simulink model "AircraftSimulation_RealTime"  (R2017a)
settings: Solver=ode45  StartTime=0.0  StopTime=inf  RelTol=1e-3  EnableMultiTasking=on
model workspace (MAT data in the model file):
  rho = Simulink.Parameter
  rho.Value = 1.225
  rho.DataType = 'auto'
  rho.Dimensions = [1 1]
values from neighbouring files (symbols this model uses):
  AR = 9.8    [ControlTuning.m]
  b = 12.8016    [ControlTuning.m]
  c = 1.3533    [ControlTuning.m]
  D = d    [rscale.m]
  m = 2521    [ControlTuning.m]
  N = inv([A,B;C,D])*Z'    [rscale.m]
  rho = 0.66    [ControlTuning.m]
  S = 16.72254    [ControlTuning.m]
  s = tf('s')    [ControlTuning.m]    (also in rscale.m = size(A,1))
  W = m*g    (= 24731.01)    [ControlTuning.m]
  Z = [zeros([1,s]) 1]    [rscale.m]
  zeta = Ix*Iz - Ixz^2    (= 5250689.81)    [ControlTuning.m]
undefined symbols (not defined in the file or in its folder): cdo, CLa, ClB, Clda, CLde, Cldr, CLmax, CLo, Clp, CLq, Clr, Cma, Cmde, Cmo, Cmq, CnB, Cnda, Cndr, Cnp, Cnr, CYB, CYda, CYdr, CYp, CYr, da, de, dr, dT, dV_x, dV_y, dV_z, elevation, h, I, Isp, mo, mu_e, springK, StallAngle, T, tblackstrip, tControl, tWind, X, xground, xland, Y, yground, yland, ZeroTolerance
libraries: sm_lib x46, nesl_utility x21, simulink x10, realtime_pacer_lib x1
(part 1 of 2)
settings Model: Creator=alexandermclean  LastModifiedBy=alexandermclean
settings SolverCC: ZeroCrossAlgorithm=Adaptive
settings DataIOCC: LimitDataPoints=on  MaxDataPoints=3000  SaveFormat=Array  SaveState=on  ReturnWorkspaceOutputs=on
settings OptimizationCC: LifeSpan=inf
settings DebuggingCC: SFUnexpectedBacktrackingDiag=warning  SFNoUnconditionalDefaultTransitionDiag=warning  SFExecutionAtInitializationDiag=none
settings HardwareCC: ProdBitPerPointer=32  ProdBitPerSizeT=32  ProdBitPerPtrDiffT=32  ProdLargestAtomicFloat=None  ProdIntDivRoundTo=Undefined  ProdEndianess=Unspecified  ProdWordSize=32  ProdHWDeviceType=32-bit Generic
settings ModelReferenceCC: PropagateSignalLabelsOutOfModel=off
settings GRTTargetCC: TargetLangStandard=C89/C90 (ANSI)  GeneratePreprocessorConditionals=Disable all
settings ConfigComp: CovMetricSettings=dw  CovHtmlReporting=on  CovSaveCumulativeToWorkspaceVar=on  CovSaveSingleToWorkspaceVar=on  CovExternalEMLEnable=off
settings ExplorerConfigSet: InternalSimMechanicsExplorerSettings="<ExplorerConfiguration><canonicalview>default</canonicalview><AnimationSetting><BasePlaybackSpeed>1.0</BasePlaybackSpeed><PlaybackSpeedFactor>1.0</PlaybackSpeedFactor></AnimationSetting><TilePanel><TileInfo><Tiles Columns=\"1\" Count=\"1\" Rows=\"1\"><Column Left=\"2\" Weight=\"1\"/><Column Left=\"358\"/><Row Top=\"2\" Weight=\"1\"/><Row Top=\"515\"/><Tile Height=\"1\" Width=\"1\" X=\"0\" Y=\"0\"/></Tiles></TileInfo><SceneInfo><SceneViewer><BGColor><R>0.200000002980232239</R><G>1</G><B>1</B></BGColor><Camera><DoPerspective>off</DoPerspective><Position><X>-5383371.51956753805</X><Y>16528461.3354325853</Y><Z>-20295565.3065634556</Z></Position><Center><X>-424001.534646867425</X><Y>1302358.08165564947</Y><Z>-1688034.52349125012</Z></Center><Up><X>0.659279124000458405</X><Y>-0.486194351728896135</Y><Z>-0.573555654670152237</Z></Up><ViewLimDist>1</ViewLimDist><YLim>4.3662398520704988e-10</YLim><XLim>3.00612148545329968e-10</XLim></Camera></SceneViewer></SceneInfo></TilePanel><MechEditorPanel><Cameras><Camera><Id>Camera1</Id><Value><Name>Driver View</Name><NativeCamera><PositionTrackingFeature>Aircraft_Simulation.Dynamics_Simscape.Drivers_View1.R</PositionTrackingFeature><CenterTrackingFeature>Aircraft_Simulation.Dynamics_Simscape.Drivers_View1.R</CenterTrackingFeature><UpVectorTrackingFeature>Aircraft_Simulation.Dynamics_Simscape.Drivers_View1.R</UpVectorTrackingFeature><CenterTrackingOrigin>off</CenterTrackingOrigin><CenterTrackingDirection>+X</CenterTrackingDirection><UpVectorTrackingDirection>+Z</UpVectorTrackingDirection></NativeCamera></Value></Camera><Camera><Id>Camera2</Id><Value><Name>Front View</Name><NativeCamera><PositionTrackingFeature>Aircraft_Simulation.Dynamics_Simscape.Front_View1.R</PositionTrackingFeature><CenterTrackingFeature>Aircraft_Simulation.Dynamics_Simscape.Front_View1.R</CenterTrackingFeature><UpVectorTrackingFeature>Aircraft_Simulation.Dynamics_Simscape.Front_View1.R</UpVectorTrackingFeature><CenterTrackingOrigin>off</CenterTrackingOrigin><CenterTrackingDirection>-Z</CenterTrackingDirection><UpVectorTrackingDirection>-X</UpVectorTrackingDirection></NativeCamera></Value></Camera><Camera><Id>Camera3</Id><Value><Name>Side View</Name><NativeCamera><PositionTrackingFeature>Aircraft_Simulation.Dynamics_Simscape.Side_View1.R</PositionTrackingFeature><CenterTrackingFeature>Aircraft_Simulation.Dynamics_Simscape.Side_View1.R</CenterTrackingFeature><UpVectorTrackingFeature>Aircraft_Simulation.Dynamics_Simscape.Side_View1.R</UpVectorTrackingFeature><CenterTrackingOrigin>off</CenterTrackingOrigin><CenterTrackingDirection>+Y</CenterTrackingDirection><UpVectorTrackingDirection>-X</UpVectorTrackingDirection></NativeCamera></Value></Camera></Cameras><GfxPanelCameraMap/><VideoCreator><PlaybackSpeedRatio>1.0</PlaybackSpeedRatio><FrameRate>30</FrameRate><VideoFormat>Motion JPEG AVI</VideoFormat><FrameSize>auto</FrameSize></VideoCreator></MechEditorPanel></ExplorerConfiguration>"

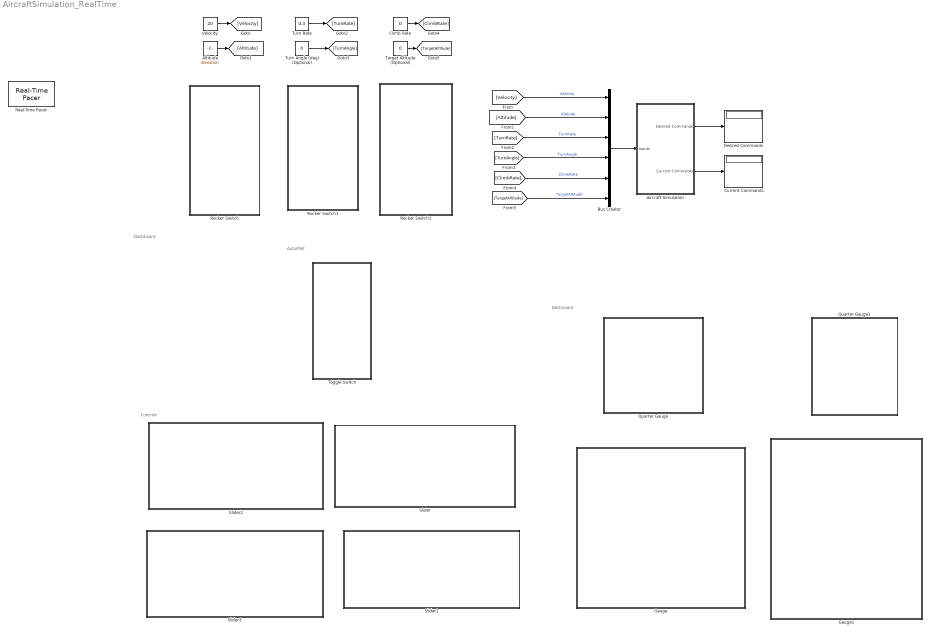
== system AircraftSimulation_RealTime ==
  note: Dashboard
  note: Controls
  note: Dashnoard
  note: AutoPilot
  Aircraft Simulation : Subsystem
  Altitude : Constant  Value=elevation
  Bus Creator : BusCreator  Inputs=6
  Climb Rate : Constant  Value=0
  Current Commands : Display
  Desired Commands : Display
  Gauge : Subsystem  DialogController=hmiCreateDDGDialog  IsWebBlock=on  mask(MWDashboardBlock){webBlockId=67f8af45-a9bd-4350-b479-67b86532381e, webBlockType=circulargauge, ShowInLibBrowser=on, ShowInitialText=on, HMISrcModelName=AircraftSimulation_RealTime}
      mask prompts: webBlockId "WebBlock Id"; webBlockType "WebBlock Type"; HMISrcModelName "Source Model"
      mask help: SimulinkHMI:dialogs:CircularGaugeDialogDesc
      mask Help: helpview([docroot '/mapfiles/simulink.map'], 'hmi_gauge')
      mask Display:
      | if strcmp(get_param(bdroot(gcb),'BlockDiagramType'), 'library')
      |     image([(matlabroot) '/toolbox/simulink/hmi/icons/CircularGauge.png']);
      | end
  Gauge1 : Subsystem  DialogController=hmiCreateDDGDialog  IsWebBlock=on  mask(MWDashboardBlock){webBlockId=380ac432-086c-412e-99f4-435f69615b16, webBlockType=circulargauge, ShowInLibBrowser=on, ShowInitialText=on, HMISrcModelName=AircraftSimulation_RealTime}
      mask prompts: webBlockId "WebBlock Id"; webBlockType "WebBlock Type"; HMISrcModelName "Source Model"
      mask help: SimulinkHMI:dialogs:CircularGaugeDialogDesc
      mask Help: helpview([docroot '/mapfiles/simulink.map'], 'hmi_gauge')
      mask Display:
      | if strcmp(get_param(bdroot(gcb),'BlockDiagramType'), 'library')
      |     image([(matlabroot) '/toolbox/simulink/hmi/icons/CircularGauge.png']);
      | end
  Quarter Gauge : Subsystem  DialogController=hmiCreateDDGDialog  IsWebBlock=on  mask(MWDashboardBlock){webBlockId=95437b06-cebb-4a55-906e-b2c61c378e79, webBlockType=ninetydegreegauge, ShowInLibBrowser=on, ShowInitialText=on, HMISrcModelName=AircraftSimulation_RealTime}
      mask prompts: webBlockId "WebBlock Id"; webBlockType "WebBlock Type"; HMISrcModelName "Source Model"
      mask help: SimulinkHMI:dialogs:NinetydegreeGaugeDialogDesc
      mask Help: helpview([docroot '/mapfiles/simulink.map'], 'hmi_quarter_gauge')
      mask Display:
      | if strcmp(get_param(bdroot(gcb),'BlockDiagramType'), 'library')
      |     image([(matlabroot) '/toolbox/simulink/hmi/icons/NinetyDegreeGauge.png']);
      | end
  Quarter Gauge1 : Subsystem  DialogController=hmiCreateDDGDialog  IsWebBlock=on  mask(MWDashboardBlock){webBlockId=bd2f9303-b0cf-4f11-bfc9-0c1a96ff53ef, webBlockType=ninetydegreegauge, ShowInLibBrowser=on, ShowInitialText=on, HMISrcModelName=AircraftSimulation_RealTime}
      mask prompts: webBlockId "WebBlock Id"; webBlockType "WebBlock Type"; HMISrcModelName "Source Model"
      mask help: SimulinkHMI:dialogs:NinetydegreeGaugeDialogDesc
      mask Help: helpview([docroot '/mapfiles/simulink.map'], 'hmi_quarter_gauge')
      mask Display:
      | if strcmp(get_param(bdroot(gcb),'BlockDiagramType'), 'library')
      |     image([(matlabroot) '/toolbox/simulink/hmi/icons/NinetyDegreeGauge.png']);
      | end
  Real-Time Pacer : realtime_pacer_lib/Real-Time Pacer  simTimePerRealTime=1
  Rocker Switch : Subsystem  DialogController=hmiCreateDDGDialog  IsWebBlock=on  mask(MWDashboardBlock){webBlockId=fc3eccde-041d-4b84-9ecd-21842f4d67ff, webBlockType=rockerswitch, ShowInLibBrowser=on, ShowInitialText=on, HMISrcModelName=AircraftSimulation_RealTime}
      mask prompts: webBlockId "WebBlock Id"; webBlockType "WebBlock Type"; HMISrcModelName "Source Model"
      mask help: SimulinkHMI:dialogs:SwitchDialogDesc
      mask Help: helpview([docroot '/mapfiles/simulink.map'], 'hmi_rocker_switch')
      mask Display:
      | if strcmp(get_param(bdroot(gcb),'BlockDiagramType'), 'library')
      |     image([(matlabroot) '/toolbox/simulink/hmi/icons/RockerSwitch.png']);
      | end
  Rocker Switch1 : Subsystem  DialogController=hmiCreateDDGDialog  IsWebBlock=on  mask(MWDashboardBlock){webBlockId=dc990da5-677e-4d98-94b9-87c965764d26, webBlockType=rockerswitch, ShowInLibBrowser=on, ShowInitialText=on, HMISrcModelName=AircraftSimulation_RealTime}
      mask prompts: webBlockId "WebBlock Id"; webBlockType "WebBlock Type"; HMISrcModelName "Source Model"
      mask help: SimulinkHMI:dialogs:SwitchDialogDesc
      mask Help: helpview([docroot '/mapfiles/simulink.map'], 'hmi_rocker_switch')
      mask Display:
      | if strcmp(get_param(bdroot(gcb),'BlockDiagramType'), 'library')
      |     image([(matlabroot) '/toolbox/simulink/hmi/icons/RockerSwitch.png']);
      | end
  Rocker Switch2 : Subsystem  DialogController=hmiCreateDDGDialog  IsWebBlock=on  mask(MWDashboardBlock){webBlockId=1b32aaf5-d39d-42dc-bc83-2804a198291e, webBlockType=rockerswitch, ShowInLibBrowser=on, ShowInitialText=on, HMISrcModelName=AircraftSimulation_RealTime}
      mask prompts: webBlockId "WebBlock Id"; webBlockType "WebBlock Type"; HMISrcModelName "Source Model"
      mask help: SimulinkHMI:dialogs:SwitchDialogDesc
      mask Help: helpview([docroot '/mapfiles/simulink.map'], 'hmi_rocker_switch')
      mask Display:
      | if strcmp(get_param(bdroot(gcb),'BlockDiagramType'), 'library')
      |     image([(matlabroot) '/toolbox/simulink/hmi/icons/RockerSwitch.png']);
      | end
  Slider : Subsystem  DialogController=hmiCreateDDGDialog  IsWebBlock=on  mask(MWDashboardBlock){webBlockId=21ec2cde-896d-490e-83b9-19082907d4f5, webBlockType=slider, ShowInLibBrowser=on, ShowInitialText=on, HMISrcModelName=AircraftSimulation_RealTime}
      mask prompts: webBlockId "WebBlock Id"; webBlockType "WebBlock Type"; HMISrcModelName "Source Model"
      mask help: SimulinkHMI:dialogs:SliderDialogDesc
      mask Help: helpview([docroot '/mapfiles/simulink.map'], 'hmi_slider')
      mask Display:
      | if strcmp(get_param(bdroot(gcb),'BlockDiagramType'), 'library')
      |     image([(matlabroot) '/toolbox/simulink/hmi/icons/Slider.png']);
      | end
  Slider1 : Subsystem  DialogController=hmiCreateDDGDialog  IsWebBlock=on  mask(MWDashboardBlock){webBlockId=1d21c48f-609f-4438-ac6a-622a61b7def2, webBlockType=slider, ShowInLibBrowser=on, ShowInitialText=on, HMISrcModelName=AircraftSimulation_RealTime}
      mask prompts: webBlockId "WebBlock Id"; webBlockType "WebBlock Type"; HMISrcModelName "Source Model"
      mask help: SimulinkHMI:dialogs:SliderDialogDesc
      mask Help: helpview([docroot '/mapfiles/simulink.map'], 'hmi_slider')
      mask Display:
      | if strcmp(get_param(bdroot(gcb),'BlockDiagramType'), 'library')
      |     image([(matlabroot) '/toolbox/simulink/hmi/icons/Slider.png']);
      | end
  Slider2 : Subsystem  DialogController=hmiCreateDDGDialog  IsWebBlock=on  mask(MWDashboardBlock){webBlockId=c2aec1fe-8232-42fd-811c-b469951ff54e, webBlockType=slider, ShowInLibBrowser=on, ShowInitialText=on, HMISrcModelName=AircraftSimulation_RealTime}
      mask prompts: webBlockId "WebBlock Id"; webBlockType "WebBlock Type"; HMISrcModelName "Source Model"
      mask help: SimulinkHMI:dialogs:SliderDialogDesc
      mask Help: helpview([docroot '/mapfiles/simulink.map'], 'hmi_slider')
      mask Display:
      | if strcmp(get_param(bdroot(gcb),'BlockDiagramType'), 'library')
      |     image([(matlabroot) '/toolbox/simulink/hmi/icons/Slider.png']);
      | end
  Slider3 : Subsystem  DialogController=hmiCreateDDGDialog  IsWebBlock=on  mask(MWDashboardBlock){webBlockId=bc4d324b-da30-4baa-91b4-3aa56de8667c, webBlockType=slider, ShowInLibBrowser=on, ShowInitialText=on, HMISrcModelName=AircraftSimulation_RealTime}
      mask prompts: webBlockId "WebBlock Id"; webBlockType "WebBlock Type"; HMISrcModelName "Source Model"
      mask help: SimulinkHMI:dialogs:SliderDialogDesc
      mask Help: helpview([docroot '/mapfiles/simulink.map'], 'hmi_slider')
      mask Display:
      | if strcmp(get_param(bdroot(gcb),'BlockDiagramType'), 'library')
      |     image([(matlabroot) '/toolbox/simulink/hmi/icons/Slider.png']);
      | end
  Target Altitude (Optional) : Constant  Value=0
  Toggle Switch : Subsystem  DialogController=hmiCreateDDGDialog  IsWebBlock=on  mask(MWDashboardBlock){webBlockId=dcb6ed43-b1b9-4957-aceb-26a4fc5c1c0a, webBlockType=toggleswitch, ShowInLibBrowser=on, ShowInitialText=on, HMISrcModelName=AircraftSimulation_RealTime}
      mask prompts: webBlockId "WebBlock Id"; webBlockType "WebBlock Type"; HMISrcModelName "Source Model"
      mask help: SimulinkHMI:dialogs:SwitchDialogDesc
      mask Help: helpview([docroot '/mapfiles/simulink.map'], 'hmi_toggle_switch')
      mask Display:
      | if strcmp(get_param(bdroot(gcb),'BlockDiagramType'), 'library')
      |     image([(matlabroot) '/toolbox/simulink/hmi/icons/ToggleSwitch.png']);
      | end
  "Turn Angle (deg) (Optional) " : Constant  Value=0
  Turn Rate : Constant  Value=0.3
  Velocity : Constant  Value=20
  wires:
  Aircraft Simulation/1(Desired Commands) -> Desired Commands/1
  Aircraft Simulation/2(Current Commands) -> Current Commands/1
  Bus Creator/1 -> Aircraft Simulation/1(Inputs)
  Velocity/1 -> [Velocity]
  Altitude/1 -> [Altitude]
  Turn Rate/1 -> [TurnRate]
  "Turn Angle (deg) (Optional) "/1 -> [TurnAngle]
  Climb Rate/1 -> [ClimbRate]
  Target Altitude (Optional)/1 -> [TargetAltitude]
  [Velocity] -> Bus Creator/1  "Velocity"
  [Altitude] -> Bus Creator/2  "Altitude"
  [TurnRate] -> Bus Creator/3  "TurnRate"
  [TurnAngle] -> Bus Creator/4  "TurnAngle"
  [ClimbRate] -> Bus Creator/5  "ClimbRate"
  [TargetAltitude] -> Bus Creator/6  "TargetAltitude"

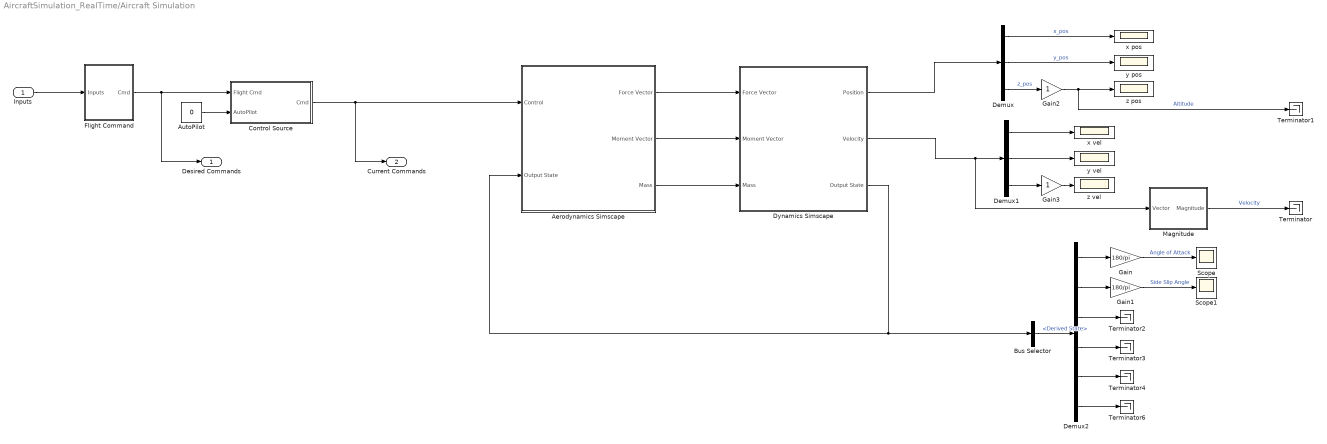
== system AircraftSimulation_RealTime/Aircraft Simulation ==
  Inputs : Inport
  Aerodynamics Simscape : Subsystem
  AutoPilot : Constant  Value=0
  Bus Selector : BusSelector  OutputSignals=Derived State
  Control Source : Subsystem
  Demux : Demux  Outputs=3
  Demux1 : Demux  Outputs=3
  Demux2 : Demux  Outputs=6
  Dynamics Simscape : Subsystem
  Flight Command : Subsystem
  Gain : Gain  Gain=180/pi
  Gain1 : Gain  Gain=180/pi
  Gain2 : Gain
  Gain3 : Gain
  Magnitude : Subsystem
  Scope : Scope
  Scope1 : Scope
  Terminator{,1..4,6} (6 alike) : Terminator
  x pos : Scope
  x vel : Scope
  y pos : Scope
  y vel : Scope
  z pos : Scope
  z vel : Scope
  Desired Commands : Outport
  Current Commands : Outport  Port=2
  wires:
  Magnitude/1(Magnitude) -> Terminator/1  "Velocity"
  Aerodynamics Simscape/1(Force Vector) -> Dynamics Simscape/1(Force Vector)
  Aerodynamics Simscape/2(Moment Vector) -> Dynamics Simscape/2(Moment Vector)
  AutoPilot/1 -> Control Source/2(AutoPilot)
  Control Source/1(Cmd) -> Current Commands/1, Aerodynamics Simscape/1(Control)
  Flight Command/1(Cmd) -> Desired Commands/1, Control Source/1(Flight Cmd)
  Demux/1 -> x pos/1  "x_pos"
  Demux/2 -> y pos/1  "y_pos"
  Demux/3 -> Gain2/1  "z_pos"
  Dynamics Simscape/3(Output State) -> Aerodynamics Simscape/2(" Output State"), Bus Selector/1
  Aerodynamics Simscape/3(Mass) -> Dynamics Simscape/3(Mass)
  Demux1/3 -> Gain3/1
  Demux1/1 -> x vel/1
  Dynamics Simscape/2(Velocity) -> Magnitude/1(Vector), Demux1/1
  Demux1/2 -> y vel/1
  Demux2/6 -> Terminator6/1
  Demux2/3 -> Terminator2/1
  Demux2/1 -> Gain/1
  Demux2/2 -> Gain1/1
  Demux2/4 -> Terminator3/1
  Dynamics Simscape/1(Position) -> Demux/1
  Bus Selector/1 -> Demux2/1  "<Derived State>"
  Demux2/5 -> Terminator4/1
  Gain1/1 -> Scope1/1  "Side Slip Angle"
  Gain/1 -> Scope/1  "Angle of Attack"
  Inputs/1 -> Flight Command/1(Inputs)
  Gain2/1 -> Terminator1/1, z pos/1  "Altitude"
  Gain3/1 -> z vel/1

== system AircraftSimulation_RealTime/Gauge ==

== system AircraftSimulation_RealTime/Gauge1 ==

== system AircraftSimulation_RealTime/Quarter Gauge ==

== system AircraftSimulation_RealTime/Quarter Gauge1 ==

== system AircraftSimulation_RealTime/Rocker Switch ==

== system AircraftSimulation_RealTime/Rocker Switch1 ==

== system AircraftSimulation_RealTime/Rocker Switch2 ==

== system AircraftSimulation_RealTime/Slider ==

== system AircraftSimulation_RealTime/Slider1 ==

== system AircraftSimulation_RealTime/Slider2 ==

== system AircraftSimulation_RealTime/Slider3 ==

== system AircraftSimulation_RealTime/Toggle Switch ==

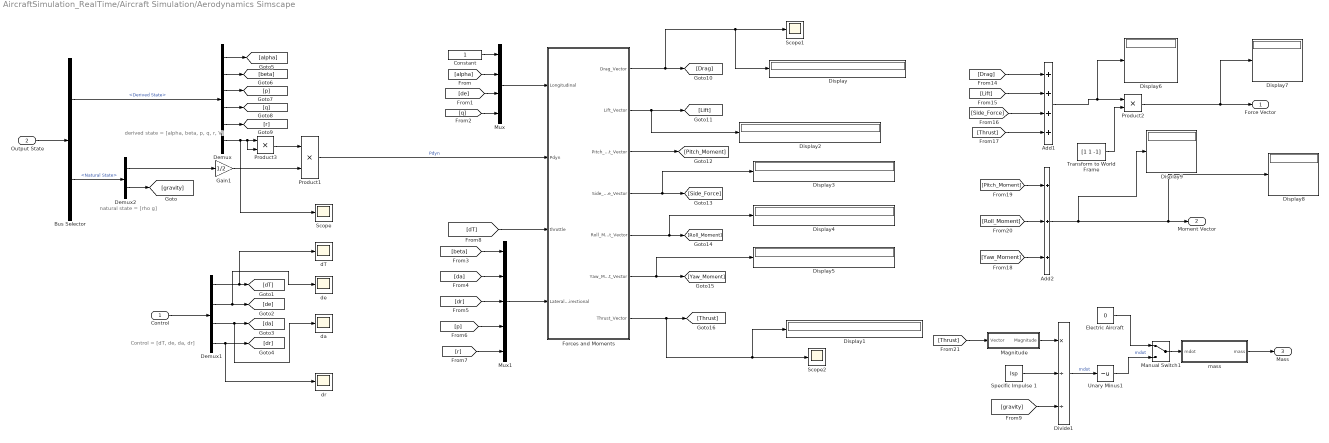
== system AircraftSimulation_RealTime/Aircraft Simulation/Aerodynamics Simscape ==
  note: Control = [dT, de, da, dr]
  note: derived state = [alpha, beta, p, q, r, V]
  note: natural state = [rho g]
  Control : Inport
  " Output State" : Inport  Port=2
  Add1 : Sum  Inputs=++++
  Add2 : Sum  Inputs=+++
  Bus Selector : BusSelector  OutputSignals=Derived State,Natural State
  Constant : Constant
  Demux : Demux  Outputs=6
  Demux1 : Demux
  Demux2 : Demux  Outputs=2
  Display{,1..9} (10 alike) : Display
  Divide1 : Product  Inputs=*//
  Electric Aircraft : Constant  Value=0
  Forces and Moments : Subsystem
  Gain1 : Gain  Gain=1/2
  Magnitude : Subsystem
  Manual Switch1 : ManualSwitch
  Mux : Mux
  Mux1 : Mux  Inputs=5
  Product1 : Product
  Product2 : Product
  Product3 : Product
  Scope : Scope
  Scope1 : Scope
  Scope2 : Scope
  Specific Impulse 1 : Constant  Value=Isp
  Transform to World Frame : Constant  Value=[1 1 -1]
  Unary Minus1 : UnaryMinus
  dT : Scope
  da : Scope
  de : Scope
  dr : Scope
  mass : Subsystem
  Force Vector : Outport
  Moment Vector : Outport  Port=2
  Mass : Outport  Port=3
  wires:
  Demux1/3 -> [da], da/1
  mass/1(mass) -> Mass/1
  Manual Switch1/1 -> mass/1(mdot)
  [dT] -> Forces and Moments/3("throttle ")
  Forces and Moments/7(Thrust_Vector) -> [Thrust], Scope2/1, Display1/1
  Forces and Moments/6(Yaw_Moment_Vector) -> [Yaw_Moment], Display5/1
  Forces and Moments/5(Roll_Moment_Vector) -> [Roll_Moment], Display4/1
  Forces and Moments/4(Side_Force_Vector) -> [Side_Force], Display3/1
  Forces and Moments/3(Pitch_Moment_Vector) -> [Pitch_Moment]
  Forces and Moments/2(Lift_Vector) -> [Lift], Display2/1
  Forces and Moments/1(Drag_Vector) -> [Drag], Scope1/1, Display/1
  Mux1/1 -> Forces and Moments/4(Lateral-Directional)
  Mux/1 -> Forces and Moments/1(Longitudinal)
  Magnitude/1(Magnitude) -> Divide1/1
  [Thrust] -> Magnitude/1(Vector)
  Electric Aircraft/1 -> Manual Switch1/1
  Unary Minus1/1 -> Manual Switch1/2  "mdot"
  [gravity] -> Divide1/3
  Divide1/1 -> Unary Minus1/1  "mdot"
  Specific Impulse 1/1 -> Divide1/2
  [Lift] -> Add1/2
  [Roll_Moment] -> Add2/2
  [Pitch_Moment] -> Add2/1
  [Yaw_Moment] -> Add2/3
  [Thrust] -> Add1/4
  [Side_Force] -> Add1/3
  [Drag] -> Add1/1
  [r] -> Mux1/5
  [beta] -> Mux1/1
  [p] -> Mux1/4
  [dr] -> Mux1/3
  [da] -> Mux1/2
  [q] -> Mux/4
  [de] -> Mux/3
  [alpha] -> Mux/2
  Constant/1 -> Mux/1
  Demux/5 -> [r]
  Demux/4 -> [q]
  Demux/3 -> [p]
  Demux/2 -> [beta]
  Demux/1 -> [alpha]
  Demux1/4 -> [dr], dr/1
  Demux1/2 -> [de], de/1
  Demux1/1 -> [dT], dT/1
  Product1/1 -> Forces and Moments/2(Pdyn)  "Pdyn"
  Gain1/1 -> Product1/2
  Demux2/2 -> [gravity]
  Product3/1 -> Product1/1
  Demux/6 -> Product3/1, Product3/2, Scope/1
  Demux2/1 -> Gain1/1
  Bus Selector/2 -> Demux2/1  "<Natural State>"
  Bus Selector/1 -> Demux/1  "<Derived State>"
  " Output State"/1 -> Bus Selector/1
  Control/1 -> Demux1/1
  Add2/1 -> Display8/1, Moment Vector/1, Display9/1
  Product2/1 -> Display7/1, Force Vector/1
  Transform to World Frame/1 -> Product2/2
  Add1/1 -> Display6/1, Product2/1

== system AircraftSimulation_RealTime/Aircraft Simulation/Control Source ==
  Flight Cmd : Inport
  AutoPilot : Inport  Port=2
  Aileron : Constant  Value=0
  Elevator : Constant  Value=0.0613138686131
  Mux : Mux
  Rudder : Constant  Value=0
  Switch : Switch  Threshold=1
  Thrust : Constant  Value=0
  Cmd : Outport
  wires:
  Switch/1 -> Cmd/1
  AutoPilot/1 -> Switch/2
  Thrust/1 -> Mux/1
  Elevator/1 -> Mux/2
  Rudder/1 -> Mux/4
  Aileron/1 -> Mux/3
  Flight Cmd/1 -> Switch/1
  Mux/1 -> Switch/3

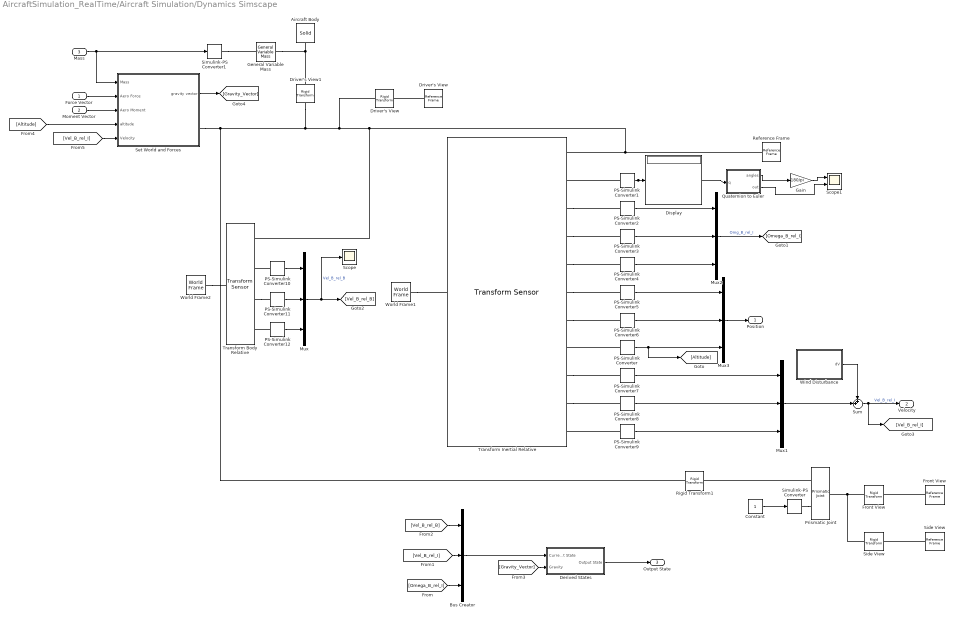
== system AircraftSimulation_RealTime/Aircraft Simulation/Dynamics Simscape ==
  Force Vector : Inport
  Moment Vector : Inport  Port=2
  Mass : Inport  Port=3
  " Driver's View" : sm_lib/Frames and Transforms/Reference Frame
  " Front View" : sm_lib/Frames and Transforms/Reference Frame
  " Side View" : sm_lib/Frames and Transforms/Reference Frame
  Aircraft Body : sm_lib/Body Elements/Solid  InertiaType=Custom  Mass=0  MassUnits=kg  CenterOfMass=[0 0 0]  CenterOfMassUnits=m  MomentsOfInertia=[0 0 0]  MomentsOfInertiaUnits=kg*m^2  ProductsOfInertia=[0 0 0]  ProductsOfInertiaUnits=kg*m^2  DensityBased=off  Density=62.38  DensityUnits=kg/m^3  DoExposeReferenceFrame=on  SerializedFrames=<Frames/>  GraphicType=FromGeometry  MarkerShape=Sphere  MarkerSize=10  GraphicVisPropType=SimpleVisualProperties  GraphicDiffuseColor=[0.5 0.5 0.5]  GraphicSpecularColor=[0.5 0.5 0.5 1.0]  GraphicAmbientColor=[0.15 0.15 0.15 1.0]  GraphicEmissiveColor=[0.0 0.0 0.0 1.0]  GraphicShininess=75  GraphicOpacity=1.0  GeometryShape=FromFile  RectangleSize=[1 1]  RectangleSizeUnits=m  BrickDimensions=[1 1 1]  BrickDimensionUnits=m  CylinderRadius=1  CylinderRadiusUnits=m  CylinderLength=1  CylinderLengthUnits=m  SphereRadius=1  SphereRadiusUnits=m  EllipsoidRadii=[1 1 1]  EllipsoidRadiiUnits=m  ExtrusionCrossSection=[1 1; -1 1; -1 -1; 1 -1]  ExtrusionCrossSectionUnits=m  ExtrusionLength=1  ExtrusionLengthUnits=m  PolygonNumSides=3  PolygonOuterRadius=1  PolygonOuterRadiusUnits=m  ExtGeomFileType=STEP  ExtGeomFileName=/Users/alexandermclean/Documents/MATLAB/BreakPlane/Rc_Aircraft v2.step  ExtGeomFileUnits=m  RevolutionCrossSection=[1 1; 1 -1; 2 -1; 2 1]  RevolutionCrossSectionUnits=m  RevolutionExtent=Full  RevolutionAngle=180  RevolutionAngleUnits=deg
  Bus Creator : BusCreator  Inputs=3
  Constant : Constant
  Derived States : Subsystem
  Display : Display
  Driver's View : sm_lib/Frames and Transforms/Rigid Transform  TranslationMethod=Cartesian  TranslationStandardOffset=0  TranslationLengthUnit=m  TranslationStandardAxis=+Z  TranslationCartesianOffset=driverView  TranslationROffset=0  TranslationROffsetUnits=m  TranslationZOffset=0  TranslationZOffsetUnits=m  TranslationThetaOffset=0  TranslationThetaOffsetUnits=deg  RotationMethod=AlignedAxes  RotationAngleUnits=deg  RotationStandardAxis=+Z  RotationAngle=0.0  RotationArbitraryAxis=[0 0 1]  FollAlignAxisA=+Z  BaseAlignAxisA=-Z  FollAlignAxisB=+X  BaseAlignAxisB=+X  RotationSequenceAxes=FollowerAxes  RotationSequence=XYX  RotationSequenceAngles=[0 0 0]  RotationSequenceAnglesUnits=deg  RotationMatrix=[1 0 0; 0 1 0; 0 0 1]
  Driver's View1 : sm_lib/Frames and Transforms/Rigid Transform  TranslationMethod=Cartesian  TranslationStandardOffset=0  TranslationLengthUnit=m  TranslationStandardAxis=+Z  TranslationCartesianOffset=driverView  TranslationROffset=0  TranslationROffsetUnits=m  TranslationZOffset=0  TranslationZOffsetUnits=m  TranslationThetaOffset=0  TranslationThetaOffsetUnits=deg  RotationMethod=AlignedAxes  RotationAngleUnits=deg  RotationStandardAxis=+Z  RotationAngle=0.0  RotationArbitraryAxis=[0 0 1]  FollAlignAxisA=-X  BaseAlignAxisA=+X  FollAlignAxisB=+Y  BaseAlignAxisB=-Z  RotationSequenceAxes=FollowerAxes  RotationSequence=XYX  RotationSequenceAngles=[0 0 0]  RotationSequenceAnglesUnits=deg  RotationMatrix=[1 0 0; 0 1 0; 0 0 1]
  "Front View " : sm_lib/Frames and Transforms/Rigid Transform  TranslationMethod=Cartesian  TranslationStandardOffset=0  TranslationLengthUnit=m  TranslationStandardAxis=+Z  TranslationCartesianOffset=frontView  TranslationROffset=0  TranslationROffsetUnits=m  TranslationZOffset=0  TranslationZOffsetUnits=m  TranslationThetaOffset=0  TranslationThetaOffsetUnits=deg  RotationMethod=None  RotationAngleUnits=deg  RotationStandardAxis=+Z  RotationAngle=0.0  RotationArbitraryAxis=[0 0 1]  FollAlignAxisA=+Z  BaseAlignAxisA=+X  FollAlignAxisB=+Y  BaseAlignAxisB=+Y  RotationSequenceAxes=FollowerAxes  RotationSequence=XYX  RotationSequenceAngles=[0 0 0]  RotationSequenceAnglesUnits=deg  RotationMatrix=[1 0 0; 0 1 0; 0 0 1]
  Gain : Gain  Gain=180/pi
  General Variable Mass : sm_lib/Body Elements/Variable Mass/General Variable Mass  VariableInertiaType=Custom  MassType=TimeVarying  Mass=1  MassUnits=kg  CenterOfMassType=Constant  CenterOfMass=[h 0 0]  CenterOfMassUnits=m  InertiaMatrixType=Constant  MomentsOfInertia=[I I I]  MomentsOfInertiaUnits=kg*m^2  ProductsOfInertia=[0 0 0]  ProductsOfInertiaUnits=kg*m^2  GraphicType=InertiaEllipsoid  MarkerShape=Sphere  MarkerSize=10  GraphicVisPropType=SimpleVisualProperties  GraphicDiffuseColor=[0 1 0]  GraphicSpecularColor=[0.5 0.5 0.5 1.0]  GraphicAmbientColor=[0.15 0.15 0.15 1.0]  GraphicEmissiveColor=[0.0 0.0 0.0 1.0]  GraphicShininess=75  GraphicOpacity=0
      settings: SourceProductName=Simscape Multibody  SourceProductBaseCode=MS
  Mux{,1..3} (4 alike) : Mux  Inputs=3
  PS-Simulink Converter{,1..12} (13 alike) : nesl_utility/PS-Simulink Converter  PhysicalDomain=network_engine_domain  SubClassName=ps_output  LeftPortType=input  RightPortType=output  PseudoPeriodic=off  Frequencies=[]  Unit=1  AffineConversion=off
  Prismatic Joint : sm_lib/Joints/Prismatic Joint  SenseConstraintForce=off  SenseConstraintForceX=off  SenseConstraintForceY=off  SenseConstraintForceZ=off  SenseConstraintTorque=off  SenseConstraintTorqueX=off  SenseConstraintTorqueY=off  SenseConstraintTorqueZ=off  SenseTotalForce=off  SenseTotalForceX=off  SenseTotalForceY=off  SenseTotalForceZ=off  SenseTotalTorque=off  SenseTotalTorqueX=off  SenseTotalTorqueY=off  SenseTotalTorqueZ=off  CompositeWrenchDir=FollowerOnBase  CompositeWrenchFrame=BaseFrame  EquilibriumPosition=0  EquilibriumPositionUnits=m  SpringStiffness=0  SpringStiffnessUnits=N/m  DampingCoefficient=0  DampingCoefficientUnits=N/(m/s)  TorqueActuationMode=ComputedTorque  MotionActuationMode=InputMotion  SensePosition=off  SenseVelocity=off  SenseAcceleration=off  SenseTorqueForce=off  PositionTargetSpecify=on  PositionTargetPriority=High  PositionTargetValue=0  PositionTargetValueUnits=m  VelocityTargetSpecify=off  VelocityTargetPriority=High  VelocityTargetValue=0  VelocityTargetValueUnits=m/s
  Quaternion to Euler : MATLAB Function  TreatAsAtomicUnit=on
  Reference Frame : sm_lib/Frames and Transforms/Reference Frame
  Rigid Transform1 : sm_lib/Frames and Transforms/Rigid Transform  TranslationMethod=None  TranslationStandardOffset=0  TranslationLengthUnit=m  TranslationStandardAxis=+Z  TranslationCartesianOffset=[0 0 0]  TranslationROffset=0  TranslationROffsetUnits=m  TranslationZOffset=0  TranslationZOffsetUnits=m  TranslationThetaOffset=0  TranslationThetaOffsetUnits=deg  RotationMethod=AlignedAxes  RotationAngleUnits=deg  RotationStandardAxis=+Z  RotationAngle=0.0  RotationArbitraryAxis=[0 0 1]  FollAlignAxisA=+Z  BaseAlignAxisA=-Z  FollAlignAxisB=+Y  BaseAlignAxisB=+Y  RotationSequenceAxes=FollowerAxes  RotationSequence=XZX  RotationSequenceAngles=[90 0 0]  RotationSequenceAnglesUnits=deg  RotationMatrix=[1 0 0; 0 1 0; 0 0 1]
  Scope : Scope
  Scope1 : Scope  NumInputPorts=2
  Set World and Forces : Subsystem
  "Side View " : sm_lib/Frames and Transforms/Rigid Transform  TranslationMethod=Cartesian  TranslationStandardOffset=0  TranslationLengthUnit=m  TranslationStandardAxis=+Z  TranslationCartesianOffset=sideView  TranslationROffset=0  TranslationROffsetUnits=m  TranslationZOffset=0  TranslationZOffsetUnits=m  TranslationThetaOffset=0  TranslationThetaOffsetUnits=deg  RotationMethod=None  RotationAngleUnits=deg  RotationStandardAxis=+Z  RotationAngle=0.0  RotationArbitraryAxis=[0 0 1]  FollAlignAxisA=+Z  BaseAlignAxisA=+X  FollAlignAxisB=+Y  BaseAlignAxisB=+Y  RotationSequenceAxes=FollowerAxes  RotationSequence=XYX  RotationSequenceAngles=[0 0 0]  RotationSequenceAnglesUnits=deg  RotationMatrix=[1 0 0; 0 1 0; 0 0 1]
  Simulink-PS Converter : nesl_utility/Simulink-PS Converter  PhysicalDomain=network_engine_domain  SubClassName=ps_input  LeftPortType=input  RightPortType=output  PseudoPeriodic=off  Frequencies=[]  NoiseDistribution=none  NoiseParameters=[]  Unit=1  AffineConversion=off  FilteringAndDerivatives=provide  SimscapeFilterOrder=1  InputFilterTimeConstant=0.001  UdotUserProvided=0
  Simulink-PS Converter1 : nesl_utility/Simulink-PS Converter  PhysicalDomain=network_engine_domain  SubClassName=ps_input  LeftPortType=input  RightPortType=output  PseudoPeriodic=off  Frequencies=[]  NoiseDistribution=none  NoiseParameters=[]  Unit=1  AffineConversion=off  FilteringAndDerivatives=provide  SimscapeFilterOrder=1  InputFilterTimeConstant=0.001  UdotUserProvided=0
  Sum : Sum  Inputs=++|
  Transform Body Relative : sm_lib/Frames and Transforms/Transform Sensor  MeasurementFrame=NonRotatingFollower  SenseAngle=off  SenseAxis=off  SenseAngle1=off  SenseAngle2=off  SenseAngle3=off  SenseQ=off  SenseR=off  SenseOmegaX=off  SenseOmegaY=off  SenseOmegaZ=off  SenseOmega1=off  SenseOmega2=off  SenseOmega3=off  SenseQDot=off  SenseRDot=off  SenseAlphaX=off  SenseAlphaY=off  SenseAlphaZ=off  SenseAlpha1=off  SenseAlpha2=off  SenseAlpha3=off  SenseQDDot=off  SenseRDDot=off  SenseX=off  SenseY=off  SenseZ=off  SenseRad=off  SenseAzim=off  SenseDist=off  SenseInc=off  SenseXDot=on  SenseYDot=on  SenseZDot=on  SenseRadDot=off  SenseAzimDot=off  SenseDistDot=off  SenseIncDot=off  SenseXDDot=off  SenseYDDot=off  SenseZDDot=off  SenseRadDDot=off  SenseAzimDDot=off  SenseDistDDot=off  SenseIncDDot=off
  Transform Inertial Relative : sm_lib/Frames and Transforms/Transform Sensor  MeasurementFrame=World  SenseAngle=off  SenseAxis=off  SenseAngle1=off  SenseAngle2=off  SenseAngle3=off  SenseQ=on  SenseR=off  SenseOmegaX=on  SenseOmegaY=on  SenseOmegaZ=on  SenseOmega1=off  SenseOmega2=off  SenseOmega3=off  SenseQDot=off  SenseRDot=off  SenseAlphaX=off  SenseAlphaY=off  SenseAlphaZ=off  SenseAlpha1=off  SenseAlpha2=off  SenseAlpha3=off  SenseQDDot=off  SenseRDDot=off  SenseX=on  SenseY=on  SenseZ=on  SenseRad=off  SenseAzim=off  SenseDist=off  SenseInc=off  SenseXDot=on  SenseYDot=on  SenseZDot=on  SenseRadDot=off  SenseAzimDot=off  SenseDistDot=off  SenseIncDot=off  SenseXDDot=off  SenseYDDot=off  SenseZDDot=off  SenseRadDDot=off  SenseAzimDDot=off  SenseDistDDot=off  SenseIncDDot=off
  Wind Disturbance : Subsystem
  World Frame1 : sm_lib/Frames and Transforms/World Frame
  World Frame2 : sm_lib/Frames and Transforms/World Frame
  Position : Outport
  Velocity : Outport  Port=2
  Output State : Outport  Port=3
  wires:
  PS-Simulink Converter5/1 -> Mux3/1
  PS-Simulink Converter6/1 -> Mux3/2
  PS-Simulink Converter8/1 -> Mux1/2
  PS-Simulink Converter7/1 -> Mux1/1
  PS-Simulink Converter2/1 -> Mux2/1
  PS-Simulink Converter3/1 -> Mux2/2
  PS-Simulink Converter4/1 -> Mux2/3
  PS-Simulink Converter1/1 -> Quaternion to Euler/1(q), Display/1
  Force Vector/1 -> Set World and Forces/2(Aero Force)
  Moment Vector/1 -> Set World and Forces/3(Aero Moment)
  PS-Simulink Converter10/1 -> Mux/1
  PS-Simulink Converter11/1 -> Mux/2
  PS-Simulink Converter12/1 -> Mux/3
  Mux/1 -> Scope/1, [Vel_B_rel_B]  "Vel_B_rel_B"
  PS-Simulink Converter9/1 -> Mux1/3
  Mux2/1 -> [Omega_B_rel_I]  "Omg_B_rel_I"
  [Omega_B_rel_I] -> Bus Creator/3
  [Vel_B_rel_I] -> Bus Creator/2
  [Vel_B_rel_B] -> Bus Creator/1
  Bus Creator/1 -> Derived States/1(Current State)
  Set World and Forces/1(gravity vector) -> [Gravity_Vector]
  [Gravity_Vector] -> Derived States/2(Gravity)
  Derived States/1(Output State) -> Output State/1
  [Altitude] -> Set World and Forces/4(altitude)
  Constant/1 -> Simulink-PS Converter/1
  Sum/1 -> [Vel_B_rel_I], Velocity/1  "Vel_B_rel_I"
  Mux1/1 -> Sum/2
  Wind Disturbance/1(dV) -> Sum/1
  Mux3/1 -> Position/1
  Mass/1 -> Set World and Forces/1(Mass), Simulink-PS Converter1/1
  [Vel_B_rel_I] -> Set World and Forces/5(Velocity)
  PS-Simulink Converter/1 -> [Altitude], Mux3/3
  Quaternion to Euler/1(angles) -> Gain/1
  Gain/1 -> Scope1/1
  Quaternion to Euler/2(out) -> Scope1/2
  connections:
  World Frame1/RConn1 -- Transform Inertial Relative/LConn1
  PS-Simulink Converter1/LConn1 -- Transform Inertial Relative/RConn2
  PS-Simulink Converter/LConn1 -- Transform Inertial Relative/RConn8
  PS-Simulink Converter9/LConn1 -- Transform Inertial Relative/RConn11
  Transform Inertial Relative/RConn10 -- PS-Simulink Converter8/LConn1
  Transform Inertial Relative/RConn9 -- PS-Simulink Converter7/LConn1
  Transform Inertial Relative/RConn7 -- PS-Simulink Converter6/LConn1
  Transform Inertial Relative/RConn6 -- PS-Simulink Converter5/LConn1
  Transform Inertial Relative/RConn5 -- PS-Simulink Converter4/LConn1
  Transform Inertial Relative/RConn4 -- PS-Simulink Converter3/LConn1
  Transform Inertial Relative/RConn3 -- PS-Simulink Converter2/LConn1
  World Frame2/RConn1 -- Transform Body Relative/LConn1
  PS-Simulink Converter10/LConn1 -- Transform Body Relative/RConn2
  PS-Simulink Converter12/LConn1 -- Transform Body Relative/RConn4
  Transform Body Relative/RConn3 -- PS-Simulink Converter11/LConn1
  Prismatic Joint/LConn1 -- Rigid Transform1/RConn1
  "Front View "/LConn1 -- "Side View "/LConn1 -- Prismatic Joint/RConn1
  " Side View"/RConn1 -- "Side View "/RConn1
  " Front View"/RConn1 -- "Front View "/RConn1
  " Driver's View"/RConn1 -- Driver's View/RConn1
  Simulink-PS Converter/RConn1 -- Prismatic Joint/LConn2
  Simulink-PS Converter1/RConn1 -- General Variable Mass/LConn1
  Set World and Forces/RConn1 -- Driver's View1/RConn1 -- Reference Frame/RConn1 -- Transform Inertial Relative/RConn1 -- Transform Body Relative/RConn1 -- Driver's View/LConn1 -- Rigid Transform1/LConn1
  General Variable Mass/RConn1 -- Driver's View1/LConn1 -- Aircraft Body/RConn1

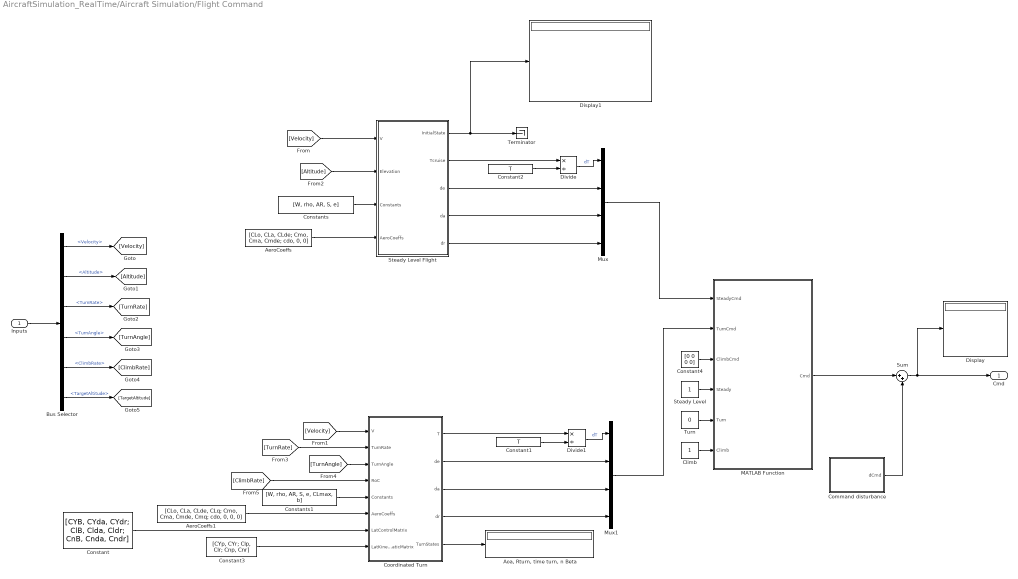
== system AircraftSimulation_RealTime/Aircraft Simulation/Flight Command ==
  Inputs : Inport
  AeroCoeffs : Constant  Value=[CLo, CLa, CLde; Cmo, Cma, Cmde; cdo, 0, 0]
  AeroCoeffs1 : Constant  Value=[CLo, CLa, CLde, CLq; Cmo, Cma, Cmde, Cmq; cdo, 0, 0, 0]
  "Aoa, Rturn, time turn, n Beta" : Display
  Bus Selector : BusSelector  OutputSignals=Velocity,Altitude,TurnRate,TurnAngle,ClimbRate,TargetAltitude
  Climb : Constant
  Command disturbance : Subsystem
  Constant : Constant  Value=[CYB, CYda, CYdr; ClB, Clda, Cldr; CnB, Cnda, Cndr]
  Constant1 : Constant  Value=T
  Constant2 : Constant  Value=T
  Constant3 : Constant  Value=[CYp, CYr; Clp, Clr; Cnp, Cnr]
  Constant4 : Constant  Value=[0 0 0 0]
  Constants : Constant  Value=[W, rho, AR, S, e]
  Constants1 : Constant  Value=[W, rho, AR, S, e, CLmax, b]
  Coordinated Turn : MATLAB Function  TreatAsAtomicUnit=on
  Display : Display
  Display1 : Display
  Divide : Product  Inputs=*/
  Divide1 : Product  Inputs=*/
  MATLAB Function : MATLAB Function  TreatAsAtomicUnit=on
  Mux : Mux
  Mux1 : Mux
  Steady Level : Constant
  "Steady Level Flight " : MATLAB Function  TreatAsAtomicUnit=on
  Sum : Sum  Inputs=|++
  Terminator : Terminator
  Turn : Constant  Value=0
  Cmd : Outport
  wires:
  [Velocity] -> "Steady Level Flight "/1(V)
  "Steady Level Flight "/1(InitialState) -> Terminator/1, Display1/1
  [Altitude] -> "Steady Level Flight "/2(Elevation)
  Constant2/1 -> Divide/2
  "Steady Level Flight "/2(Tcruise) -> Divide/1
  "Steady Level Flight "/3(de) -> Mux/2
  "Steady Level Flight "/4(da) -> Mux/3
  "Steady Level Flight "/5(dr) -> Mux/4
  Divide/1 -> Mux/1  "dT"
  Constants/1 -> "Steady Level Flight "/3(Constants)
  AeroCoeffs/1 -> "Steady Level Flight "/4(AeroCoeffs)
  Sum/1 -> Display/1, Cmd/1
  Command disturbance/1(dCmd) -> Sum/2
  Divide1/1 -> Mux1/1  "dT"
  Constants1/1 -> Coordinated Turn/5(Constants)
  Coordinated Turn/3(da) -> Mux1/3
  Coordinated Turn/2(de) -> Mux1/2
  [Velocity] -> Coordinated Turn/1(V)
  Constant1/1 -> Divide1/2
  Coordinated Turn/4(dr) -> Mux1/4
  AeroCoeffs1/1 -> Coordinated Turn/6(AeroCoeffs)
  Coordinated Turn/1(T) -> Divide1/1
  Mux1/1 -> MATLAB Function/2(TurnCmd)
  Constant/1 -> Coordinated Turn/7(LatControlMatrix)
  Constant3/1 -> Coordinated Turn/8(LatKinematicMatrix)
  Coordinated Turn/5(TurnStates) -> "Aoa, Rturn, time turn, n Beta"/1
  [TurnRate] -> Coordinated Turn/2(TurnRate)
  Inputs/1 -> Bus Selector/1
  Bus Selector/1 -> [Velocity]  "<Velocity>"
  Bus Selector/2 -> [Altitude]  "<Altitude>"
  Bus Selector/3 -> [TurnRate]  "<TurnRate>"
  Bus Selector/4 -> [TurnAngle]  "<TurnAngle>"
  [TurnAngle] -> Coordinated Turn/3(TurnAngle)
  Bus Selector/5 -> [ClimbRate]  "<ClimbRate>"
  [ClimbRate] -> Coordinated Turn/4(RoC)
  Bus Selector/6 -> [TargetAltitude]  "<TargetAltitude>"
  Mux/1 -> MATLAB Function/1(SteadyCmd)
  Steady Level/1 -> MATLAB Function/4(Steady)
  Climb/1 -> MATLAB Function/6(Climb)
  Turn/1 -> MATLAB Function/5(Turn)
  Constant4/1 -> MATLAB Function/3(ClimbCmd)
  MATLAB Function/1(Cmd) -> Sum/1

== system AircraftSimulation_RealTime/Aircraft Simulation/Magnitude ==
  Vector : Inport
  Demux : Demux  Outputs=3
  Product1 : Product
  Product2 : Product
  Product3 : Product
  Sqrt : Sqrt  SaturateOnIntegerOverflow=on
  Sum : Sum  Inputs=+++
  Magnitude : Outport
  wires:
  Demux/1 -> Product1/1, Product1/2
  Demux/3 -> Product3/1, Product3/2
  Product2/1 -> Sum/2
  Product1/1 -> Sum/1
  Sum/1 -> Sqrt/1
  Demux/2 -> Product2/1, Product2/2
  Product3/1 -> Sum/3
  Vector/1 -> Demux/1
  Sqrt/1 -> Magnitude/1

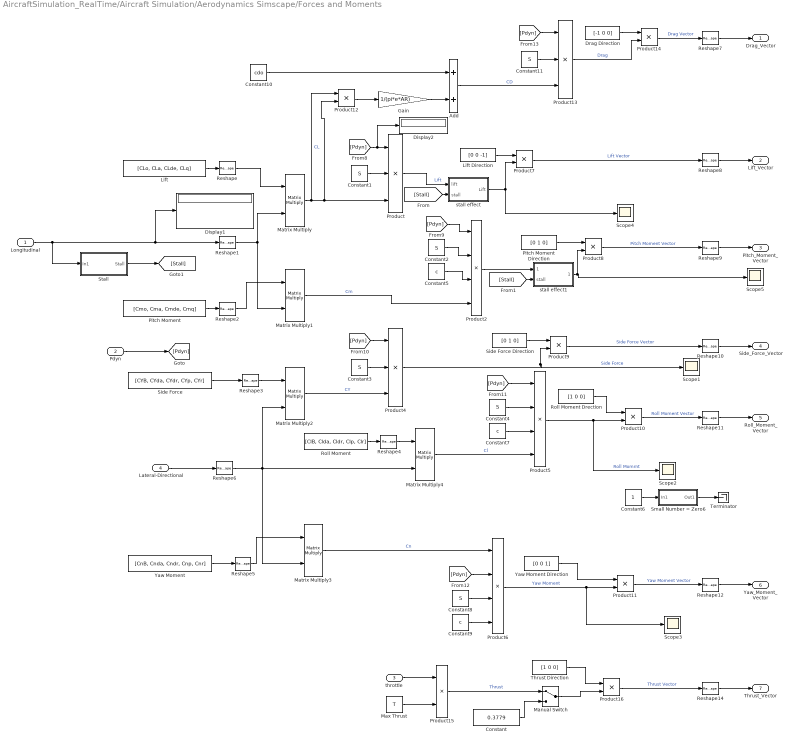
== system AircraftSimulation_RealTime/Aircraft Simulation/Aerodynamics Simscape/Forces and Moments ==
  Longitudinal : Inport
  Pdyn : Inport  Port=2
  "throttle " : Inport  Port=3
  Lateral-Directional : Inport  Port=4
  Add : Sum
  Constant : Constant  Value=0.3779
  Constant{1..4,8,11} (6 alike) : Constant  Value=S
  Constant10 : Constant  Value=cdo
  Constant5 : Constant  Value=c
  Constant6 : Constant
  Constant7 : Constant  Value=c
  Constant9 : Constant  Value=c
  Display1 : Display
  Display2 : Display
  Drag Direction : Constant  Value=[-1 0 0]
  Gain : Gain  Gain=1/(pi*e*AR)
  Lift : Constant  Value=[CLo, CLa, CLde, CLq]
  Lift Direction : Constant  Value=[0 0 -1]
  Manual Switch : ManualSwitch
  Matrix Multiply{,1..4} (5 alike) : Product  Multiplication=Matrix(*)
  Max Thrust : Constant  Value=T
  Pitch Moment : Constant  Value=[Cmo, Cma, Cmde, Cmq]
  Pitch Moment Direction : Constant  Value=[0 1 0]
  Product : Product  Inputs=3
  Product{7..12,14..16} (9 alike) : Product
  Product13 : Product  Inputs=3
  Product2 : Product  Inputs=4
  Product4 : Product  Inputs=3
  Product5 : Product  Inputs=4
  Product6 : Product  Inputs=4
  Reshape{,2..5} (5 alike) : Reshape  OutputDimensionality=Row vector (2-D)
  Reshape{1,6..12,14} (9 alike) : Reshape  OutputDimensionality=Column vector (2-D)
  Roll Moment : Constant  Value=[ClB, Clda, Cldr, Clp, Clr]
  "Roll Moment Drection " : Constant  Value=[1 0 0]
  Scope{1..5} (5 alike) : Scope
  Side Force : Constant  Value=[CYB, CYda, CYdr, CYp, CYr]
  Side Force Direction : Constant  Value=[0 1 0]
  Small Number = Zero6 : Subsystem
  Stall : Subsystem
  Terminator : Terminator
  Thrust Direction : Constant  Value=[1 0 0]
  Yaw Moment : Constant  Value=[CnB, Cnda, Cndr, Cnp, Cnr]
  Yaw Moment Direction : Constant  Value=[0 0 1]
  stall effect : Subsystem
  stall effect1 : Subsystem
  Drag_Vector : Outport
  Lift_Vector : Outport  Port=2
  Pitch_Moment_Vector : Outport  Port=3
  Side_Force_Vector : Outport  Port=4
  Roll_Moment_Vector : Outport  Port=5
  Yaw_Moment_Vector : Outport  Port=6
  Thrust_Vector : Outport  Port=7
  wires:
  Small Number = Zero6/1(Out1) -> Terminator/1
  Constant6/1 -> Small Number = Zero6/1(In1)
  Matrix Multiply4/1 -> Product5/4  "Cl"
  Reshape14/1 -> Thrust_Vector/1
  Reshape12/1 -> Yaw_Moment_Vector/1
  Reshape11/1 -> Roll_Moment_Vector/1
  Reshape10/1 -> Side_Force_Vector/1
  Reshape9/1 -> Pitch_Moment_Vector/1
  Reshape8/1 -> Lift_Vector/1
  Reshape7/1 -> Drag_Vector/1
  Manual Switch/1 -> Product16/2
  Product15/1 -> Manual Switch/1  "Thrust"
  Constant/1 -> Manual Switch/2
  Pdyn/1 -> [Pdyn]
  [Pdyn] -> Product4/1
  "throttle "/1 -> Product15/1
  Add/1 -> Product13/3  "CD"
  [Pdyn] -> Product5/1
  Constant7/1 -> Product5/3
  Reshape4/1 -> Matrix Multiply4/1
  Constant5/1 -> Product2/3
  Product8/1 -> Reshape9/1  "Pitch Moment Vector"
  Drag Direction/1 -> Product14/1
  Constant4/1 -> Product5/2
  "Roll Moment Drection "/1 -> Product10/1
  Gain/1 -> Add/2
  Product6/1 -> Product11/2, Scope3/1  "Yaw Moment"
  Product11/1 -> Reshape12/1  "Yaw Moment Vector"
  Roll Moment/1 -> Reshape4/1
  Yaw Moment Direction/1 -> Product11/1
  Lift/1 -> Reshape/1
  Reshape5/1 -> Matrix Multiply3/1
  [Pdyn] -> Product2/1
  Constant1/1 -> Product/2
  Matrix Multiply1/1 -> Product2/4  "Cm"
  Lateral-Directional/1 -> Reshape6/1
  Constant2/1 -> Product2/2
  Yaw Moment/1 -> Reshape5/1
  Constant11/1 -> Product13/2
  [Pdyn] -> Product/1, Display2/1
  [Pdyn] -> Product13/1
  Lift Direction/1 -> Product7/1
  Product12/1 -> Gain/1
  Product13/1 -> Product14/2  "Drag"
  [Pdyn] -> Product6/2
  Reshape3/1 -> Matrix Multiply2/1
  Max Thrust/1 -> Product15/2
  Reshape1/1 -> Matrix Multiply1/2, Matrix Multiply/2
  Reshape/1 -> Matrix Multiply/1
  Longitudinal/1 -> Stall/1(In1), Reshape1/1, Display1/1
  Constant3/1 -> Product4/2
  Pitch Moment/1 -> Reshape2/1
  Matrix Multiply2/1 -> Product4/3  "CY"
  Constant8/1 -> Product6/3
  Thrust Direction/1 -> Product16/1
  Matrix Multiply/1 -> Product12/1, Product/3, Product12/2  "CL"
  Product7/1 -> Reshape8/1  "Lift Vector"
  Product4/1 -> Product9/2, Scope1/1  "Side Force"
  Pitch Moment Direction/1 -> Product8/1
  Side Force Direction/1 -> Product9/1
  Constant10/1 -> Add/1
  Product5/1 -> Product10/2, Scope2/1  "Roll Momrnt"
  Product16/1 -> Reshape14/1  "Thrust Vector"
  Matrix Multiply3/1 -> Product6/1  "Cn"
  Constant9/1 -> Product6/4
  Product10/1 -> Reshape11/1  "Roll Moment Vector"
  Reshape6/1 -> Matrix Multiply2/2, Matrix Multiply4/2, Matrix Multiply3/2
  Product9/1 -> Reshape10/1  "Side Force Vector"
  Side Force/1 -> Reshape3/1
  Reshape2/1 -> Matrix Multiply1/1
  Product14/1 -> Reshape7/1  "Drag Vector"
  Stall/1(Stall) -> [Stall]
  stall effect/1(Lift) -> Scope4/1, Product7/2
  [Stall] -> stall effect/2(stall)
  Product/1 -> stall effect/1(lift)  "Lift"
  Product2/1 -> stall effect1/1(moment)
  stall effect1/1(Moment) -> Scope5/1, Product8/2
  [Stall] -> stall effect1/2(stall)

== system AircraftSimulation_RealTime/Aircraft Simulation/Aerodynamics Simscape/Magnitude ==
  Vector : Inport
  Demux : Demux  Outputs=3
  Product1 : Product
  Product2 : Product
  Product3 : Product
  Sqrt : Sqrt  SaturateOnIntegerOverflow=on
  Sum : Sum  Inputs=+++
  Magnitude : Outport
  wires:
  Sqrt/1 -> Magnitude/1
  Vector/1 -> Demux/1
  Product3/1 -> Sum/3
  Demux/2 -> Product2/2, Product2/1
  Sum/1 -> Sqrt/1
  Product1/1 -> Sum/1
  Product2/1 -> Sum/2
  Demux/3 -> Product3/2, Product3/1
  Demux/1 -> Product1/2, Product1/1

== system AircraftSimulation_RealTime/Aircraft Simulation/Aerodynamics Simscape/mass ==
  mdot : Inport
  Add : Sum
  Integrator : Integrator
  inital mass : Constant  Value=mo
  mass : Outport
  wires:
  inital mass/1 -> Add/2
  Integrator/1 -> Add/1
  mdot/1 -> Integrator/1
  Add/1 -> mass/1  "current mass"

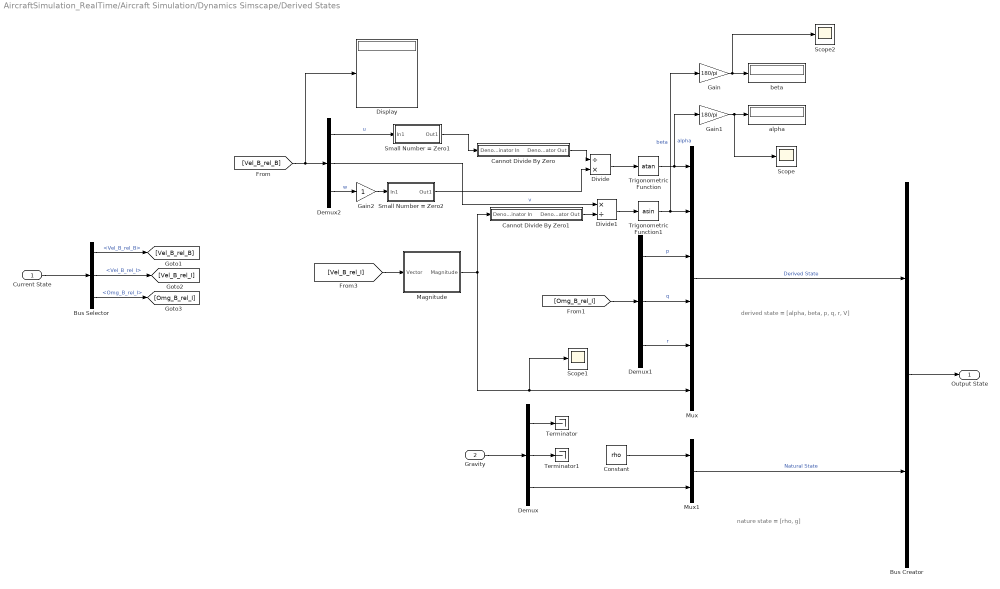
== system AircraftSimulation_RealTime/Aircraft Simulation/Dynamics Simscape/Derived States ==
  note: nature state = [rho, g]
  note: derived state = [alpha, beta, p, q, r, V]
  Current State : Inport
  Gravity : Inport  Port=2
  Bus Creator : BusCreator  Inputs=2
  Bus Selector : BusSelector  OutputSignals=Vel_B_rel_B,Vel_B_rel_I,Omg_B_rel_I
  Cannot Divide By Zero : Subsystem
  Cannot Divide By Zero1 : Subsystem
  Constant : Constant  Value=rho
  Demux : Demux  Outputs=3
  Demux1 : Demux  Outputs=3
  Demux2 : Demux  Outputs=3
  Display : Display
  Divide : Product  Inputs=/*
  Divide1 : Product  Inputs=*/
  Gain : Gain  Gain=180/pi
  Gain1 : Gain  Gain=180/pi
  Gain2 : Gain
  Magnitude : Subsystem
  Mux : Mux  Inputs=6
  Mux1 : Mux  Inputs=2
  Scope : Scope
  Scope1 : Scope
  Scope2 : Scope
  Small Number = Zero1 : Subsystem
  Small Number = Zero2 : Subsystem
  Terminator : Terminator
  Terminator1 : Terminator
  Trigonometric Function : Trigonometry  Operator=atan
  Trigonometric Function1 : Trigonometry  Operator=asin
  alpha : Display
  beta : Display
  Output State : Outport
  wires:
  Current State/1 -> Bus Selector/1
  Bus Selector/1 -> [Vel_B_rel_B]  "<Vel_B_rel_B>"
  Bus Selector/3 -> [Omg_B_rel_I]  "<Omg_B_rel_I>"
  [Omg_B_rel_I] -> Demux1/1
  Demux1/3 -> Mux/5  "r"
  Demux1/2 -> Mux/4  "q"
  Demux1/1 -> Mux/3  "p"
  Trigonometric Function/1 -> Gain1/1, Mux/1  "alpha"
  Divide1/1 -> Trigonometric Function1/1
  Divide/1 -> Trigonometric Function/1
  Demux2/2 -> Divide1/1  "v"
  Mux1/1 -> Bus Creator/2  "Natural State"
  Bus Creator/1 -> Output State/1
  Magnitude/1(Magnitude) -> Cannot Divide By Zero1/1(Denominator In), Scope1/1, Mux/6
  [Vel_B_rel_B] -> Display/1, Demux2/1
  Trigonometric Function1/1 -> Gain/1, Mux/2  "beta"
  Mux/1 -> Bus Creator/1  "Derived State"
  Cannot Divide By Zero/1(Denominator Out) -> Divide/1
  Demux2/1 -> Small Number = Zero1/1(In1)  "u"
  Cannot Divide By Zero1/1(Denominator Out) -> Divide1/2
  Gain/1 -> Scope2/1, beta/1
  Gain1/1 -> Scope/1, alpha/1
  Bus Selector/2 -> [Vel_B_rel_I]  "<Vel_B_rel_I>"
  [Vel_B_rel_I] -> Magnitude/1(Vector)
  Demux2/3 -> Gain2/1  "w"
  Constant/1 -> Mux1/1
  Demux/1 -> Terminator/1
  Demux/2 -> Terminator1/1
  Gravity/1 -> Demux/1
  Demux/3 -> Mux1/2
  Gain2/1 -> Small Number = Zero2/1(In1)
  Small Number = Zero2/1(Out1) -> Divide/2
  Small Number = Zero1/1(Out1) -> Cannot Divide By Zero/1(Denominator In)
